simulink model "orbital_dynamics"  (R2025b)
settings: Solver=VariableStepAuto  StartTime=0.0  StopTime=10.0  RelTol=1e-3
InitFcn:
  | initialize
values from neighbouring files (symbols this model uses):
  mu = 3.986004418e14    (= 398600441800000)    [initialize_orbital_dynamics.m]
  r0 = [r0_mag; 0; 0]    [initialize_orbital_dynamics.m]
  v0 = [0; v0_mag; 0]    [initialize_orbital_dynamics.m]
undefined symbols (not defined in the file or in its folder): G, M_Earth
settings Model: Creator=jennaparker  LastModifiedBy=jennaparker

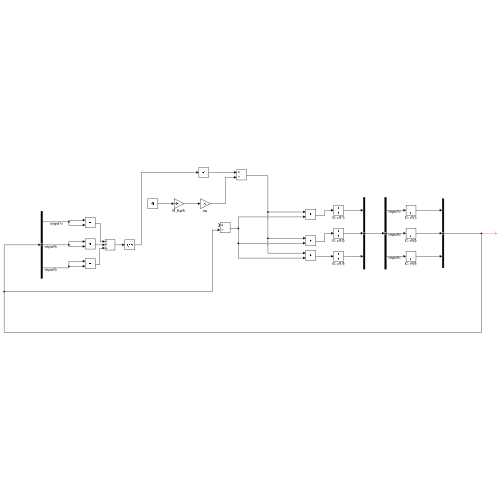
[thumbnail: Simulink's stored preview of the top-level diagram]
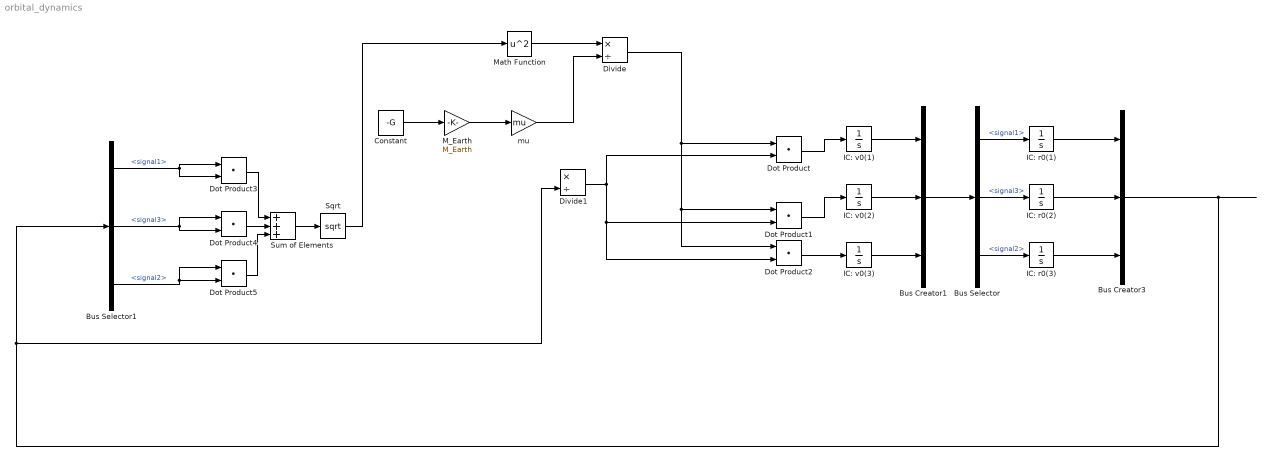
== system orbital_dynamics ==
  Bus Creator1 : BusCreator  Inputs=3
  Bus Creator3 : BusCreator  Inputs=3
  Bus Selector : BusSelector  OutputSignals=signal1,signal3,signal2
  Bus Selector1 : BusSelector  OutputSignals=signal1,signal3,signal2
  Constant : Constant  Value=-G
  Divide : Product  Inputs=*/
  Divide1 : Product  Inputs=*/
  Dot Product{,1..5} (6 alike) : DotProduct  OutDataTypeStr=Inherit: Inherit via internal rule
  IC: r0(1) : Integrator  InitialCondition=r0(1)
  IC: r0(2) : Integrator  InitialCondition=r0(2)
  IC: r0(3) : Integrator  InitialCondition=r0(3)
  IC: v0(1) : Integrator  InitialCondition=v0(1)
  IC: v0(2) : Integrator  InitialCondition=v0(2)
  IC: v0(3) : Integrator  InitialCondition=v0(3)
  M_Earth : Gain  Gain=M_Earth
  Math Function : Math  Operator=square
  Sqrt : Sqrt
  Sum of Elements : Sum  Inputs=+++
  mu : Gain  Gain=mu
  wires:
  mu/1 -> Divide/2
  Math Function/1 -> Divide/1
  Dot Product/1 -> IC: v0(1)/1
  IC: v0(1)/1 -> Bus Creator1/1
  Divide1/1 -> Dot Product2/2, Dot Product1/2, Dot Product/2
  IC: r0(3)/1 -> Bus Creator3/3
  Bus Selector1/2 -> Dot Product4/1, Dot Product4/2  "<signal3>"
  Dot Product2/1 -> IC: v0(3)/1
  IC: r0(1)/1 -> Bus Creator3/1
  Divide/1 -> Dot Product2/1, Dot Product1/1, Dot Product/1
  Bus Selector1/1 -> Dot Product3/2, Dot Product3/1  "<signal1>"
  Bus Creator3/1 -> Divide1/2, Bus Selector1/1
  Bus Selector/1 -> IC: r0(1)/1  "<signal1>"
  M_Earth/1 -> mu/1
  Bus Selector/2 -> IC: r0(2)/1  "<signal3>"
  Constant/1 -> M_Earth/1
  Bus Selector/3 -> IC: r0(3)/1  "<signal2>"
  IC: r0(2)/1 -> Bus Creator3/2
  Sum of Elements/1 -> Sqrt/1
  Dot Product4/1 -> Sum of Elements/2
  Dot Product5/1 -> Sum of Elements/3
  Bus Selector1/3 -> Dot Product5/1, Dot Product5/2  "<signal2>"
  Sqrt/1 -> Math Function/1
  Dot Product3/1 -> Sum of Elements/1
  Bus Creator1/1 -> Bus Selector/1
  IC: v0(2)/1 -> Bus Creator1/2
  Dot Product1/1 -> IC: v0(2)/1
  IC: v0(3)/1 -> Bus Creator1/3
